simulink library "NexteerUtilities"  (R2013b)
settings: Solver=FixedStepDiscrete  StartTime=0.0  StopTime=10.0  FixedStep=.1  RelTol=1e-3
undefined symbols (not defined in the file or in its folder): CF_Uls_f32, LPF_Str
libraries: NexteerUtilities x5
settings Model: Creator=mmcbroom  LastModifiedBy=DZ1YRM

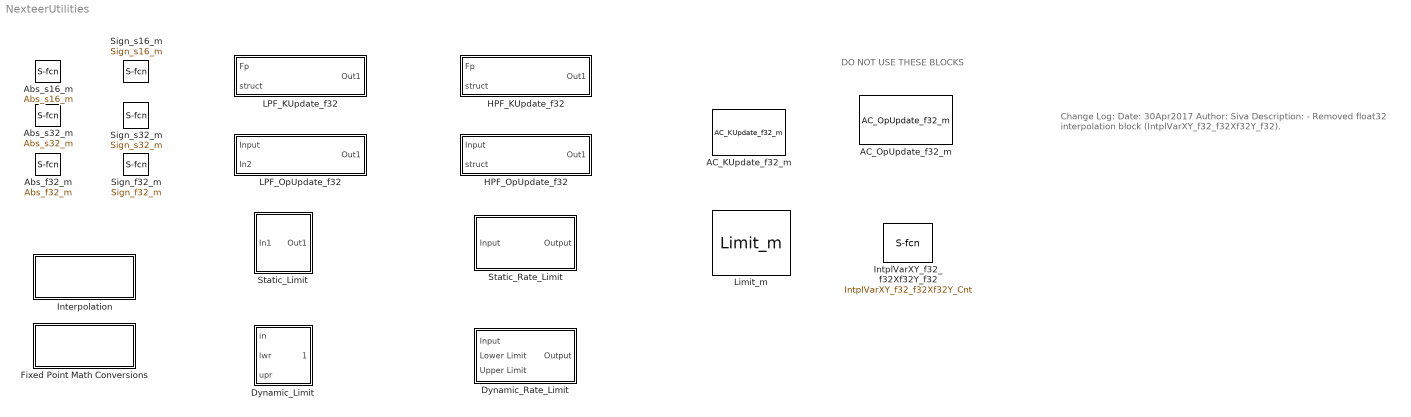
== system NexteerUtilities ==
  note: DO NOT USE THESE BLOCKS
  note: Change Log:
      |
      | Date: 30Apr2017
      | Author: Siva
      | Description:
      |      -  Removed float32 interpolation block (IntplVarXY_f32_f32Xf32Y_f32).
  AC_KUpdate_f32_m : S-Function  FunctionName=AC_KUpdate_f32_m  EnableBusSupport=off  mask(Legacy Function){}
      mask help:
      | This block allows you to call the legacy functions specified by the following Legacy Code Tool definition:
      | def.SFunctionName = 'util_LPF_KUpdate_f32';
      | def.OutputFcnSpec = 'single y1 = LPF_KUpdate_f32_m(single u1, single u2)';
      | def.HeaderFiles = {'utility.h'};
      | def.SourceFiles = {'utility.c'};
      settings: AttributesFormatString=Filt_KUpdate_f32
      mask Help: <p>This block was generated automatically by the Legacy Code Tool. For detailed help on this tool, call<a href="matlab:legacy_code('help')"> legacy_code('help')</a>.</p>
      mask Display:
      | port_label('input',1,'Fp');
      | port_label('input',2,'T');
      | port_label('output',1,'K');
      | 
      | text(0.3,0.5,'Do Not\n Use\nThis Block')
  AC_OpUpdate_f32_m : S-Function  FunctionName=AC_OpUpdate_f32_m  EnableBusSupport=off
      mask Display:
      | port_label('input',1,'in')
      | port_label('input',2,'PrevOut')
      | port_label('input',3,'K')
      | 
      | port_label('output',1,'out')
      | 
      | text(0.45,0.5,'Do Not\n Use\nThis Block')
  Abs_f32_m : S-Function  FunctionName=Abs_f32_m  EnableBusSupport=off  mask(Abs_f32){}
      mask help:
      | This block allows you to call the legacy functions specified by the following Legacy Code Tool definition:
      | def.SFunctionName = 'util_abs_f32';
      | def.OutputFcnSpec = 'single y1 = Abs_f32_m(single u1)';
      | def.HeaderFiles = {'utility.h'};
      settings: AttributesFormatString=Abs_f32
      mask Help: <p>This block was generated automatically by the Legacy Code Tool. For detailed help on this tool, call<a href="matlab:legacy_code('help')"> legacy_code('help')</a>.</p>
      mask Display:
      | fprintf('|u|');
      | %port_label('input',1,'U');
      | %port_label('output',1,'Y');
  Abs_s16_m : S-Function  FunctionName=Abs_s16_m  EnableBusSupport=off  mask(Abs_s16){}
      mask help:
      | This block allows you to call the legacy functions specified by the following Legacy Code Tool definition:
      | def.SFunctionName = 'util_abs_s16';
      | def.OutputFcnSpec = 'uint16 y1 = Abs_s16_m(int16 u1)';
      | def.HeaderFiles = {'utility.h'};
      settings: AttributesFormatString=Abs_s16
      mask Help: <p>This block was generated automatically by the Legacy Code Tool. For detailed help on this tool, call<a href="matlab:legacy_code('help')"> legacy_code('help')</a>.</p>
      mask Display:
      | fprintf('|u|');
      | %port_label('input',1,'s16');
      | %port_label('output',1,'Y');
  Abs_s32_m : S-Function  FunctionName=Abs_s32_m  EnableBusSupport=off  mask(Abs_s32){}
      mask help:
      | This block allows you to call the legacy functions specified by the following Legacy Code Tool definition:
      | def.SFunctionName = 'util_abs_s32';
      | def.OutputFcnSpec = 'uint32 y1 = Abs_s32_m(int32 u1)';
      | def.HeaderFiles = {'utility.h'};
      settings: AttributesFormatString=Abs_s32
      mask Help: <p>This block was generated automatically by the Legacy Code Tool. For detailed help on this tool, call<a href="matlab:legacy_code('help')"> legacy_code('help')</a>.</p>
      mask Display:
      | fprintf('|u|');
      | %port_label('input',1,'U');
      | %port_label('output',1,'Y');
  Dynamic_Limit : Subsystem  mask(Dynamic_Limit){}
      mask help: Simulink implementation of the Limit_m macro. This implementation allows the user to dynamically change the limit values.
      mask Display:
      | horizX = [0.2 0.9];
      | horizY = [0.55 0.55];
      | 
      | vertX = [0.55 0.55];
      | vertY = [0.2 0.8];
      | 
      | x = [.25, .35, .75, .85];
      | y = [.2, .2, .8, .8];
      | 
      | plot(horizX,horizY, vertX,vertY, x,y);
      | 
      | text(0.5,0.9,'f32', 'horizontalAlignment', 'center')
  Dynamic_Rate_Limit : Subsystem  mask(Dynamic_Rate_Limit){Ts=0}
      mask prompts: Ts "Time Step"
      mask help: Dynamic_Rate_Limit is a rate limiter with dynamic bounds.
      settings: AttributesFormatString=Time Step: %<Ts>
  Fixed Point Math Conversions : Subsystem
  HPF_KUpdate_f32 : Subsystem  mask(HPF_KUpdate_f32){Ts=0}
      mask prompts: Ts "Time Step"
      mask help: Simulink implementation of the HPF_KUpdate_f32_m macro.
      settings: AttributesFormatString=Time Step: %<Ts>
      mask Display:
      | port_label('input',1,'Hz');
      | port_label('input',2,'HPF_Str In');
      | port_label('output',1,'HPF_Str Out');
  HPF_OpUpdate_f32 : Subsystem  mask(HPF_OpUpdate_f32){}
      mask help: Simulink implementation of the HPF_OpUpdate_f32_m macro.
      mask Display:
      | port_label('input',1,'Input')
      | port_label('input',2,'HPF_Str In')
      | port_label('output',1,'HPF_Str Out')
  Interpolation : Subsystem
  IntplVarXY_f32_f32Xf32Y_f32 : S-Function  FunctionName=IntplVarXY_f32_f32Xf32Y_Cnt  Parameters=SParameter1, SParameter2  EnableBusSupport=off  mask(IntplVarXY_f32_f32Xf32Y_f32){SParameter1=ones([1 1 ]), SParameter2=ones([1 1 ])}
      mask prompts: SParameter1 "XTable:"; SParameter2 "YTable:"
      mask help:
      | This block allows you to call the legacy functions specified by the following Legacy Code Tool definition:
      | def.SFunctionName = 'IntplVarXY_f32_f32Xf32Y_Cnt';
      | def.OutputFcnSpec = 'single y1 = IntplVarXY_f32_f32Xf32Y_Cnt(single p1[], single p2[], uint16 size(p1,1), single u1)';
      | def.HeaderFiles = {'GlobalMacro.h'};
      | def.SourceFiles = {'utility.c'};
      settings: AttributesFormatString=IntplVarXY (float32)
      mask Help: <p>This block was generated automatically by the Legacy Code Tool. For detailed help on this tool, call<a href="matlab:legacy_code('help')"> legacy_code('help')</a>.</p>
      mask Display:
      | fprintf('float32\n\nInterpolate')
      | 
      | Xx = [0.1, .9];
      | Xy = [0.5, 0.5];
      | Yx = [0.5, 0.5];
      | Yy = [0.1, .8];
      | 
      | px = [.1, .3, .6, .7, .8, .9];
      | py = [.34,  .35, .39, .4, .5, .8];
      | plot(Xx,Xy, Yx,Yy, px,py)
  LPF_KUpdate_f32 : Subsystem  mask(LPF_KUpdate_f32){Ts=0}
      mask prompts: Ts "Time Step:"
      mask help: Simulink implementation of the LPF_KUpdate_f32_m macro.
      settings: AttributesFormatString=Time Step: %<Ts>
      mask Display:
      | port_label('input',1,'Hz');
      | port_label('input',2,'LPF_Str In');
      | port_label('output',1,'LPF_Str Out');
  LPF_OpUpdate_f32 : Subsystem  mask(LPF_OpUpdate_f32){}
      mask help: Simulink implementation of the LPF_OpUpdate_f32_m macro.
      mask Display:
      | port_label('input',1,'Input')
      | port_label('input',2,'LPF_Str In')
      | port_label('output',1,'LPF_Str Out')
  Limit_m : S-Function  FunctionName=Limit_m  EnableBusSupport=off
      mask help:
      | This block is being deprecated.
      | Use the Static_Limit or Dynamic_Limit blocks instead.
      settings: AttributesFormatString=%<Description>
      mask Display:
      | port_label('input',1,'U');
      | port_label('input',2,'Lower Limit');
      | port_label('input',3,'Upper Limit');
      | port_label('output',1,'Y');
      | text(0.3,0.76,'Do Not Use\nThis Block')
  Sign_f32_m : S-Function  FunctionName=Sign_f32_m  EnableBusSupport=off  mask(Sign_f32){}
      mask help:
      | This block allows you to call the legacy functions specified by the following Legacy Code Tool definition:
      | def.SFunctionName = 'util_sign_f32';
      | def.OutputFcnSpec = 'single y1 = Sign_f32_m(single u1)';
      | def.HeaderFiles = {'utility.h'};
      settings: AttributesFormatString=Sign_f32
      mask Help: <p>This block was generated automatically by the Legacy Code Tool. For detailed help on this tool, call<a href="matlab:legacy_code('help')"> legacy_code('help')</a>.</p>
      mask Display:
      | %port_label('input',1,'U');
      | %port_label('output',1,'Y');
      | 
      | Xx = [-1, 1];
      | Xy = [ 0, 0];
      | Yx = [ 0, 0];
      | Yy = [-1, 1];
      | 
      | px = [-.8, 0, 0, 0.8];
      | py = [-.4, -.4, .4, .4];
      | plot(Xx,Xy, Yx,Yy, px,py)
  Sign_s16_m : S-Function  FunctionName=Sign_s16_m  EnableBusSupport=off  mask(Sign_s16){}
      mask help:
      | This block allows you to call the legacy functions specified by the following Legacy Code Tool definition:
      | def.SFunctionName = 'util_sign_s16';
      | def.OutputFcnSpec = 'int16 y1 = Sign_s16_m(int16 u1)';
      | def.HeaderFiles = {'utility.h'};
      settings: AttributesFormatString=Sign_s16
      mask Help: <p>This block was generated automatically by the Legacy Code Tool. For detailed help on this tool, call<a href="matlab:legacy_code('help')"> legacy_code('help')</a>.</p>
      mask Display:
      | %port_label('input',1,'U');
      | %port_label('output',1,'Out');
      | 
      | Xx = [-1, 1];
      | Xy = [ 0, 0];
      | Yx = [ 0, 0];
      | Yy = [-1, 1];
      | 
      | px = [-.8, 0, 0, 0.8];
      | py = [-.4, -.4, .4, .4];
      | plot(Xx,Xy, Yx,Yy, px,py)
  Sign_s32_m : S-Function  FunctionName=Sign_s32_m  EnableBusSupport=off  mask(Sign_s32){}
      mask help:
      | This block allows you to call the legacy functions specified by the following Legacy Code Tool definition:
      | def.SFunctionName = 'util_sign_s32';
      | def.OutputFcnSpec = 'int32 y1 = Sign_s32_m(int32 u1)';
      | def.HeaderFiles = {'utility.h'};
      settings: AttributesFormatString=Sign_s32
      mask Help: <p>This block was generated automatically by the Legacy Code Tool. For detailed help on this tool, call<a href="matlab:legacy_code('help')"> legacy_code('help')</a>.</p>
      mask Display:
      | %port_label('input',1,'U');
      | %port_label('output',1,'Y');
      | 
      | Xx = [-1, 1];
      | Xy = [ 0, 0];
      | Yx = [ 0, 0];
      | Yy = [-1, 1];
      | 
      | px = [-.8, 0, 0, 0.8];
      | py = [-.4, -.4, .4, .4];
      | plot(Xx,Xy, Yx,Yy, px,py)
  Static_Limit : Subsystem  mask(Static_Limit){uprlim=0, lwrlim=0}
      mask prompts: uprlim "Upper Limit"; lwrlim "Lower Limit"
      mask help: Simulink implementation of the Limit_m macro. This implementation fixes limit values.
      settings: AttributesFormatString=|
      | Upper Limit:%<uprlim>
      | Lower Limit:%<lwrlim>
      mask Display:
      | horizX = [0.2 0.9];
      | horizY = [0.55 0.55];
      | 
      | vertX = [0.55 0.55];
      | vertY = [0.2 0.8];
      | 
      | x = [.25, .35, .75, .85];
      | y = [.2, .2, .8, .8];
      | 
      | plot(horizX,horizY, vertX,vertY, x,y);
      | 
      | text(0.5,0.9,'f32', 'horizontalAlignment', 'center')
  Static_Rate_Limit : Subsystem  mask(Static_Rate_Limit){Ts=0, LowerLimit=0, UpperLimit=0}
      mask prompts: Ts "Time Step"; LowerLimit "Lower Limit"; UpperLimit "Upper Limit"
      mask help: Static_Rate_Limit provides a rate limiter with static limit bounds.
      settings: AttributesFormatString=|
      | Time Step: %<Ts>
      | Lower Limit: %<LowerLimit>
      | Upper Limit: %<UpperLimit>

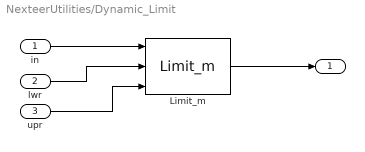
== system NexteerUtilities/Dynamic_Limit ==
  in : Inport
  lwr : Inport  Port=2
  upr : Inport  Port=3
  Limit_m : NexteerUtilities/Static_Limit/Limit_m
  " " : Outport
  wires:
  Limit_m/1 -> " "/1
  in/1 -> Limit_m/1
  lwr/1 -> Limit_m/2
  upr/1 -> Limit_m/3

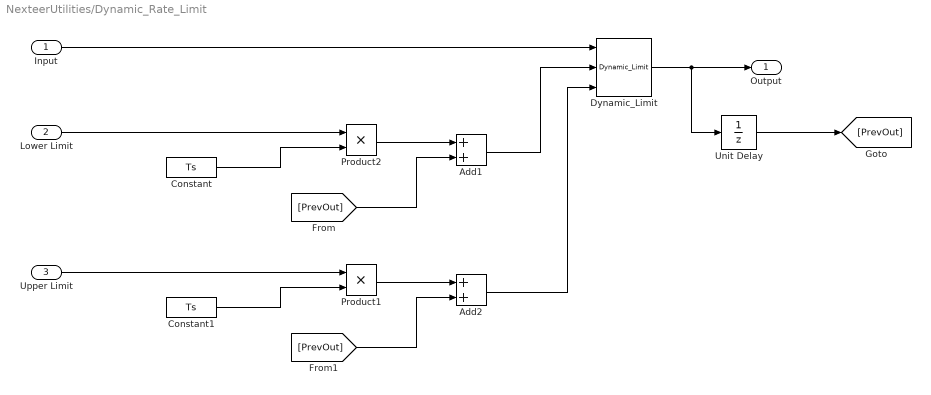
== system NexteerUtilities/Dynamic_Rate_Limit ==
  Input : Inport
  Lower Limit : Inport  Port=2
  Upper Limit : Inport  Port=3
  Add1 : Sum
  Add2 : Sum
  Constant : Constant  Value=Ts
  Constant1 : Constant  Value=Ts
  Dynamic_Limit : NexteerUtilities/Dynamic_Limit
  Product1 : Product
  Product2 : Product
  Unit Delay : UnitDelay  SampleTime=-1
  Output : Outport
  wires:
  Dynamic_Limit/1 -> Unit Delay/1, Output/1
  Input/1 -> Dynamic_Limit/1
  Constant/1 -> Product2/2
  Lower Limit/1 -> Product2/1
  Product2/1 -> Add1/1
  Unit Delay/1 -> [PrevOut]
  [PrevOut] -> Add1/2
  Constant1/1 -> Product1/2
  Upper Limit/1 -> Product1/1
  Product1/1 -> Add2/1
  [PrevOut] -> Add2/2
  Add1/1 -> Dynamic_Limit/2
  Add2/1 -> Dynamic_Limit/3

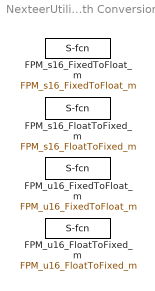
== system NexteerUtilities/Fixed Point Math Conversions ==
  FPM_s16_FixedToFloat_m : S-Function  FunctionName=FPM_s16_FixedToFloat_m  Parameters=SParameter1  EnableBusSupport=off  mask(s16_FixedToFloat){SFunctionSpec=single y1 = FPM_s16_FixedToFloat_m(int16 u1,  single p1), Param1=1}
      mask prompts: Param1 "P1:"
      mask help:
      | This block allows you to call the legacy functions specified by the following Legacy Code Tool definition:
      | def.SFunctionName = 'FPM_s16_FixedToFloat_m';
      | def.OutputFcnSpec = 'single y1 = FPM_s16_FixedToFloat_m(int16 u1,  single p1)';
      | def.HeaderFiles = {'GlobalMacro.h', 'fixmath.h'};
      | def.SourceFiles = {'utility.c'};
      | def.IncPaths = {'..'};
      | def.SrcPaths = {'..'};
      mask init:
      | SParameter1 = 2^-Param1;
      settings: AttributesFormatString=s16_FixedToFloat
      mask Help: <p>This block was generated automatically by the Legacy Code Tool. For detailed help on this tool, call<a href="matlab:legacy_code('help')"> legacy_code('help')</a>.</p>
      mask Display:
      | pnum = Param1;
      | unum = 15-Param1;
      | 
      | port_label('output',1,'f32')
      | 
      | if pnum<0
      |    fptxt = ['s' num2str(unum) 'pm' num2str(abs(pnum))];
      |    %fprintf(['s' num2str(unum) 'pm' num2str(abs(pnum))]);
      | elseif pnum>15
      |    fptxt = ['sm' num2str(abs(unum)) 'p' num2str(pnum)];
      |    %fprintf(['sm' num2str(abs(unum)) 'p' num2str(pnum)]);
      | else
      |    fptxt = ['s' num2str(unum) 'p' num2str(pnum)];
      |    %fprintf(['s' num2str(unum) 'p' num2str(pnum)]);
      | end
      | 
      | port_label('input',1,fptxt)
  FPM_s16_FloatToFixed_m : S-Function  FunctionName=FPM_s16_FloatToFixed_m  Parameters=SParameter1  EnableBusSupport=off  mask(s16_FloatToFixed){SFunctionSpec=int16  y1 = FPM_s16_FloatToFixed_m(single u1, single p1), Param1=1}
      mask prompts: Param1 "P1:"
      mask help:
      | This block allows you to call the legacy functions specified by the following Legacy Code Tool definition:
      | def.SFunctionName = 'FPM_s16_FloatToFixed_m';
      | def.OutputFcnSpec = 'int16  y1 = FPM_s16_FloatToFixed_m(single u1, single p1)';
      | def.HeaderFiles = {'GlobalMacro.h', 'fixmath.h'};
      | def.SourceFiles = {'utility.c'};
      | def.IncPaths = {'..'};
      | def.SrcPaths = {'..'};
      mask init:
      | SParameter1 = 2^Param1;
      settings: AttributesFormatString=s16_FloatToFixed
      mask Help: <p>This block was generated automatically by the Legacy Code Tool. For detailed help on this tool, call<a href="matlab:legacy_code('help')"> legacy_code('help')</a>.</p>
      mask Display:
      | pnum = Param1;
      | unum = 15-Param1;
      | 
      | port_label('input',1,'f32')
      | 
      | if pnum<0
      |     fptxt = ['s' num2str(unum) 'pm' num2str(abs(pnum))];
      |     %fprintf(['s' num2str(unum) 'pm' num2str(abs(pnum))]);
      | elseif pnum>15
      |     fptxt = ['sm' num2str(abs(unum)) 'p' num2str(pnum)];
      |     %fprintf(['sm' num2str(abs(unum)) 'p' num2str(pnum)]);
      | else
      |     fptxt = ['s' num2str(unum) 'p' num2str(pnum)];
      |     %fprintf(['s' num2str(unum) 'p' num2str(pnum)]);
      | end
      | 
      | port_label('output',1,fptxt)
  FPM_u16_FixedToFloat_m : S-Function  FunctionName=FPM_u16_FixedToFloat_m  Parameters=SParameter1  EnableBusSupport=off  mask(u16_FixedToFloat){SFunctionSpec=single y1 = FPM_u16_FixedToFloat_m(uint16 u1, single p1), Param1=1}
      mask prompts: Param1 "P1:"
      mask help:
      | This block allows you to call the legacy functions specified by the following Legacy Code Tool definition:
      | def.SFunctionName = 'FPM_u16_FixedToFloat_m';
      | def.OutputFcnSpec = 'single y1 = FPM_u16_FixedToFloat_m(uint16 u1, single p1)';
      | def.HeaderFiles = {'GlobalMacro.h', 'fixmath.h'};
      | def.SourceFiles = {'utility.c'};
      | def.IncPaths = {'..'};
      | def.SrcPaths = {'..'};
      mask init:
      | SParameter1 = 2^-Param1;
      settings: AttributesFormatString=u16_FixedToFloat
      mask Help: <p>This block was generated automatically by the Legacy Code Tool. For detailed help on this tool, call<a href="matlab:legacy_code('help')"> legacy_code('help')</a>.</p>
      mask Display:
      | pnum = Param1;
      | unum = 16-Param1;
      | 
      | port_label('output',1,'f32')
      | 
      | if pnum<0
      |    fptxt =  ['u' num2str(unum) 'pm' num2str(abs(pnum))];
      |    %fprintf(['u' num2str(unum) 'pm' num2str(abs(pnum))]);
      | elseif pnum>16
      |    fptxt = ['um' num2str(abs(unum)) 'p' num2str(pnum)];
      |    %fprintf(['um' num2str(abs(unum)) 'p' num2str(pnum)]);
      | else
      |    fptxt = ['u' num2str(unum) 'p' num2str(pnum)];
      |    %fprintf(['u' num2str(unum) 'p' num2str(pnum)]);
      | end
      | 
      | port_label('input',1,fptxt)
  FPM_u16_FloatToFixed_m : S-Function  FunctionName=FPM_u16_FloatToFixed_m  Parameters=SParameter1  EnableBusSupport=off  mask(u16_FloatToFixed){SFunctionSpec=uint16 y1 = FPM_u16_FloatToFixed_m(single u1, single p1), Param1=1}
      mask prompts: Param1 "P1:"
      mask help:
      | This block allows you to call the legacy functions specified by the following Legacy Code Tool definition:
      | def.SFunctionName = 'FPM_u16_FloatToFixed_m';
      | def.OutputFcnSpec = 'uint16 y1 = FPM_u16_FloatToFixed_m(single u1, single p1)';
      | def.HeaderFiles = {'GlobalMacro.h', 'fixmath.h'};
      | def.SourceFiles = {'utility.c'};
      | def.IncPaths = {'..'};
      | def.SrcPaths = {'..'};
      mask init:
      | SParameter1 = 2^Param1;
      settings: AttributesFormatString=u16_FloatToFixed
      mask Help: <p>This block was generated automatically by the Legacy Code Tool. For detailed help on this tool, call<a href="matlab:legacy_code('help')"> legacy_code('help')</a>.</p>
      mask Display:
      | pnum = Param1;
      | 
      | unum = 16-Param1;
      | 
      | port_label('input',1,'f32')
      | 
      | if pnum<0
      |     fptxt = ['u' num2str(unum) 'pm' num2str(abs(pnum))];
      |     %fprintf(['f32 ---> ' 'u' num2str(unum) 'pm' num2str(abs(pnum))]);
      | elseif pnum>16
      |     fptxt = ['um' num2str(abs(unum)) 'p' num2str(pnum)];
      |     %fprintf(['f32 ---> ' 'um' num2str(abs(unum)) 'p' num2str(pnum)]);
      | else
      |     fptxt = ['u' num2str(unum) 'p' num2str(pnum)];
      |     %fprintf(['f32 ---> ' 'u' num2str(unum) 'p' num2str(pnum)]);
      | end
      | 
      | port_label('output',1,fptxt)

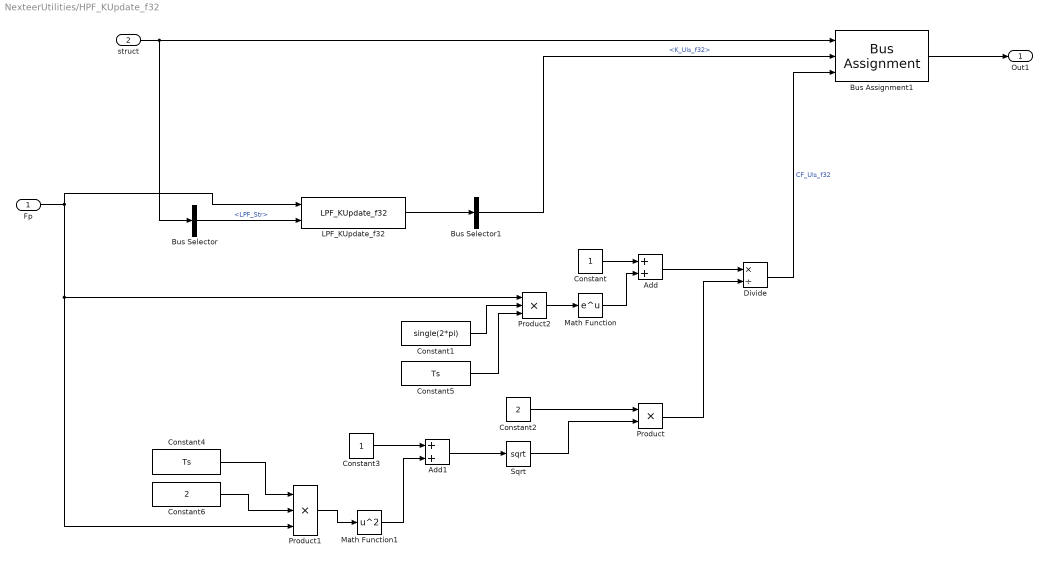
== system NexteerUtilities/HPF_KUpdate_f32 ==
  Fp : Inport
  struct : Inport  Port=2  OutDataTypeStr=Bus: HPF32KSV_Str
  Add : Sum
  Add1 : Sum
  Bus Assignment1 : BusAssignment  AssignedSignals=LPF_Str.K_Uls_f32,CF_Uls_f32
  Bus Selector : BusSelector  OutputSignals=LPF_Str
  Bus Selector1 : BusSelector  OutputSignals=K_Uls_f32
  Constant : Constant  OutDataTypeStr=single
  Constant1 : Constant  Value=single(2*pi)  OutDataTypeStr=single
  Constant2 : Constant  Value=2  OutDataTypeStr=single
  Constant3 : Constant  OutDataTypeStr=single
  Constant4 : Constant  Value=Ts  OutDataTypeStr=single
  Constant5 : Constant  Value=Ts  OutDataTypeStr=single
  Constant6 : Constant  Value=2  OutDataTypeStr=single
  Divide : Product  Inputs=*/
  LPF_KUpdate_f32 : NexteerUtilities/LPF_KUpdate_f32  Ts=Ts
  Math Function : Math  SaturateOnIntegerOverflow=on
  Math Function1 : Math  Operator=square  SaturateOnIntegerOverflow=on
  Product : Product
  Product1 : Product  Inputs=3
  Product2 : Product  Inputs=3
  Sqrt : Sqrt  SaturateOnIntegerOverflow=on
  Out1 : Outport  OutDataTypeStr=Bus: HPF32KSV_Str
  wires:
  Fp/1 -> LPF_KUpdate_f32/1, Product1/3, Product2/1
  struct/1 -> Bus Selector/1, Bus Assignment1/1
  Constant/1 -> Add/1
  Constant1/1 -> Product2/2
  Math Function/1 -> Add/2
  Add/1 -> Divide/1
  Sqrt/1 -> Product/2
  Constant2/1 -> Product/1
  Constant3/1 -> Add1/1
  Add1/1 -> Sqrt/1
  Constant4/1 -> Product1/1
  Product/1 -> Divide/2
  Product2/1 -> Math Function/1
  Math Function1/1 -> Add1/2
  Product1/1 -> Math Function1/1
  Bus Assignment1/1 -> Out1/1
  LPF_KUpdate_f32/1 -> Bus Selector1/1
  Divide/1 -> Bus Assignment1/3  "CF_Uls_f32"
  Bus Selector/1 -> LPF_KUpdate_f32/2  "<LPF_Str>"
  Bus Selector1/1 -> Bus Assignment1/2  "<K_Uls_f32>"
  Constant5/1 -> Product2/3
  Constant6/1 -> Product1/2

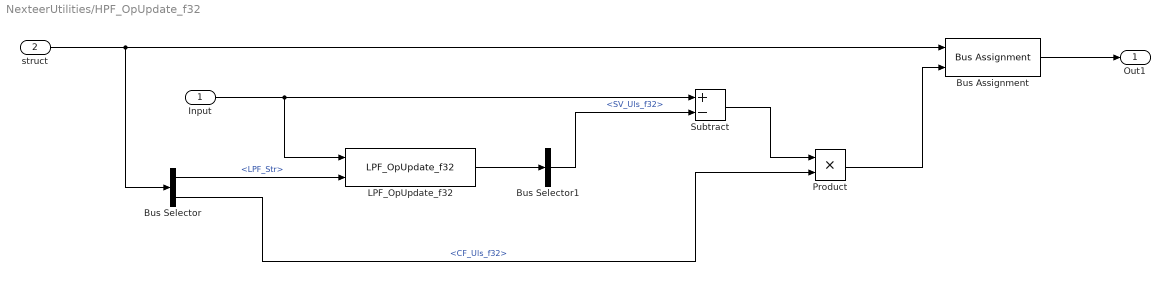
== system NexteerUtilities/HPF_OpUpdate_f32 ==
  Input : Inport
  struct : Inport  Port=2  OutDataTypeStr=Bus: HPF32KSV_Str
  Bus Assignment : BusAssignment  AssignedSignals=LPF_Str.SV_Uls_f32
  Bus Selector : BusSelector  OutputSignals=LPF_Str,CF_Uls_f32
  Bus Selector1 : BusSelector  OutputSignals=SV_Uls_f32
  LPF_OpUpdate_f32 : NexteerUtilities/LPF_OpUpdate_f32
  Product : Product
  Subtract : Sum  Inputs=+-
  Out1 : Outport  OutDataTypeStr=Bus: HPF32KSV_Str
  wires:
  struct/1 -> Bus Selector/1, Bus Assignment/1
  Bus Selector/1 -> LPF_OpUpdate_f32/2  "<LPF_Str>"
  LPF_OpUpdate_f32/1 -> Bus Selector1/1
  Input/1 -> LPF_OpUpdate_f32/1, Subtract/1
  Bus Selector1/1 -> Subtract/2  "<SV_Uls_f32>"
  Bus Selector/2 -> Product/2  "<CF_Uls_f32>"
  Subtract/1 -> Product/1
  Product/1 -> Bus Assignment/2
  Bus Assignment/1 -> Out1/1

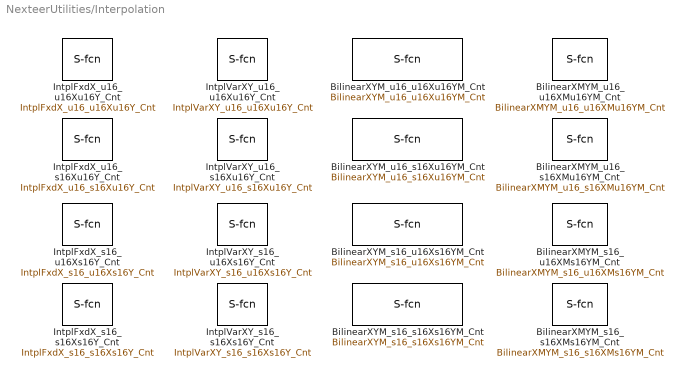
== system NexteerUtilities/Interpolation ==
  BilinearXMYM_s16_s16XMs16YM_Cnt : S-Function  FunctionName=BilinearXMYM_s16_s16XMs16YM_Cnt  Parameters=Param1,Param2,Param3  EnableBusSupport=off  mask(BilinearXMYM_s16_s16XMs16YM_Cnt){Param1=0, Param2=0, Param3=0}
      mask prompts: Param1 "BSTable:"; Param2 "XMTable:"; Param3 "YMTable:"
      settings: AttributesFormatString=Bilinear (sXM, sYM)
      mask Help: <p>This block was generated automatically by the Legacy Code Tool. For detailed help on this tool, call<a href="matlab:legacy_code('help')"> legacy_code('help')</a>.</p>
      mask Display:
      | port_label('input',1,'BS');
      | port_label('input',2,'u');
      | %port_label('output',1,'y');
      | 
      | Xx = [0.1, .9];
      | Xy = [0.5, 0.5];
      | Yx = [0.5, 0.5];
      | Yy = [0.1, .9];
      | 
      | px = [.15, .3, .6, .7, .8, .9];
      | py1 = [.1,  .1, .3, .4, .5, .9];
      | py2 = py1+0.15;
      | py3 = py2+0.15;
      | plot(Xx,Xy, Yx,Yy, px,py1, px,py2, px,py3)
  BilinearXMYM_s16_u16XMs16YM_Cnt : S-Function  FunctionName=BilinearXMYM_s16_u16XMs16YM_Cnt  Parameters=Param1,Param2,Param3  EnableBusSupport=off  mask(BilinearXMYM_s16_u16XMs16YM_Cnt){Param1=0, Param2=0, Param3=0}
      mask prompts: Param1 "BSTable:"; Param2 "XMTable:"; Param3 "YMTable:"
      settings: AttributesFormatString=Bilinear (uXM, sXM)
      mask Help: <p>This block was generated automatically by the Legacy Code Tool. For detailed help on this tool, call<a href="matlab:legacy_code('help')"> legacy_code('help')</a>.</p>
      mask Display:
      | port_label('input',1,'BS');
      | port_label('input',2,'u');
      | %port_label('output',1,'y');
      | 
      | Xx = [0.2, .9];
      | Xy = [0.4, 0.4];
      | Yx = [0.2, 0.2];
      | Yy = [0, .7];
      | 
      | px = [0.2, .3, .4, .6, .8, .9];
      | py1 = [.72, .7, .6, .3, .25, .25];
      | py2 = py1-0.1;
      | py3 = py2-0.1;
      | 
      | plot(Xx,Xy, Yx,Yy, px,py1, px,py2, px,py3)
  BilinearXMYM_u16_s16XMu16YM_Cnt : S-Function  FunctionName=BilinearXMYM_u16_s16XMu16YM_Cnt  Parameters=Param1,Param2,Param3  EnableBusSupport=off  mask(BilinearXMYM_u16_s16XMu16YM_Cnt){Param1=0, Param2=0, Param3=0}
      mask prompts: Param1 "BSTable:"; Param2 "XMTable:"; Param3 "YMTable:"
      settings: AttributesFormatString=Bilinear (sXM, uYM)
      mask Help: <p>This block was generated automatically by the Legacy Code Tool. For detailed help on this tool, call<a href="matlab:legacy_code('help')"> legacy_code('help')</a>.</p>
      mask Display:
      | port_label('input',1,'BS');
      | port_label('input',2,'u');
      | %port_label('output',1,'y');
      | 
      | Xx = [0, .9];
      | Xy = [.05, .05];
      | Yx = [.45, .45];
      | Yy = [.05, .9];
      | 
      | px = [0.15, .3, .4, .6, .7, .9];
      | py1 = [.1, .1, .2, .5, .6, .65];
      | py2 = py1+.15;
      | py3 = py2+.15;
      | 
      | plot(Xx,Xy, Yx,Yy, px,py1, px,py2, px,py3)
  BilinearXMYM_u16_u16XMu16YM_Cnt : S-Function  FunctionName=BilinearXMYM_u16_u16XMu16YM_Cnt  Parameters=Param1,Param2,Param3  EnableBusSupport=off  mask(BilinearXMYM_u16_u16XMu16YM_Cnt){Param1=0, Param2=0, Param3=0}
      mask prompts: Param1 "BSTable:"; Param2 "XMTable:"; Param3 "YMTable:"
      settings: AttributesFormatString=Bilinear (uXM, uYM)
      mask Help: <p>This block was generated automatically by the Legacy Code Tool. For detailed help on this tool, call<a href="matlab:legacy_code('help')"> legacy_code('help')</a>.</p>
      mask Display:
      | port_label('input',1,'BS');
      | port_label('input',2,'u');
      | %port_label('output',1,'y');
      | 
      | Xx = [0.2, .9];
      | Xy = [0.1, 0.1];
      | Yx = [0.2, 0.2];
      | Yy = [0.1, .7];
      | 
      | px = [0.2, .3, .4, .5, .6, .7, .9];
      | 
      | py1 = [0.1,  0.4, .6, .7, .75, .8, .8];
      | py2 = [0.1,  0.4, .5, .6, .65, .7, .7];
      | py3 = [0.1,  0.3, .4, .5, .55, .6, .6];
      | 
      | plot(Xx,Xy, Yx,Yy, px,py1, px,py2, px,py3)
  BilinearXYM_s16_s16Xs16YM_Cnt : S-Function  FunctionName=BilinearXYM_s16_s16Xs16YM_Cnt  Parameters=Param1,Param2,Param3  EnableBusSupport=off  mask(BilinearXYM_s16_s16Xs16YM_Cnt){Param1=0, Param2=0, Param3=0}
      mask prompts: Param1 "BSTable:"; Param2 "XTable:"; Param3 "YMTable:"
      settings: AttributesFormatString=Bilinear (sX, xYM)
      mask Help: <p>This block was generated automatically by the Legacy Code Tool. For detailed help on this tool, call<a href="matlab:legacy_code('help')"> legacy_code('help')</a>.</p>
      mask Display:
      | port_label('input',1,'BS');
      | port_label('input',2,'u');
      | %port_label('output',1,'y');
      | 
      | fprintf('   Bilinear Interp\n   X-tbl: s16 vector\n   Y-tbl: s16 matrix')
  BilinearXYM_s16_u16Xs16YM_Cnt : S-Function  FunctionName=BilinearXYM_s16_u16Xs16YM_Cnt  Parameters=Param1,Param2,Param3  EnableBusSupport=off  mask(BilinearXYM_s16_u16Xs16YM_Cnt){Param1=0, Param2=0, Param3=0}
      mask prompts: Param1 "BSTable:"; Param2 "XTable:"; Param3 "YMTable:"
      settings: AttributesFormatString=Bilinear (uX, sYM)
      mask Help: <p>This block was generated automatically by the Legacy Code Tool. For detailed help on this tool, call<a href="matlab:legacy_code('help')"> legacy_code('help')</a>.</p>
      mask Display:
      | port_label('input',1,'BS');
      | port_label('input',2,'u');
      | %port_label('output',1,'y');
      | 
      | fprintf('   Bilinear Interp\n   X-tbl: u16 vector\n   Y-tbl: s16 matrix')
  BilinearXYM_u16_s16Xu16YM_Cnt : S-Function  FunctionName=BilinearXYM_u16_s16Xu16YM_Cnt  Parameters=Param1,Param2,Param3  EnableBusSupport=off  mask(BilinearXYM_u16_s16Xu16YM_Cnt){Param1=0, Param2=0, Param3=0}
      mask prompts: Param1 "BSTable:"; Param2 "XTable:"; Param3 "YMTable:"
      settings: AttributesFormatString=Bilinear (sX, uYM)
      mask Help: <p>This block was generated automatically by the Legacy Code Tool. For detailed help on this tool, call<a href="matlab:legacy_code('help')"> legacy_code('help')</a>.</p>
      mask Display:
      | port_label('input',1,'BS');
      | port_label('input',2,'u');
      | %port_label('output',1,'y');
      | 
      | fprintf('   Bilinear Interp\n   X-tbl: s16 vector\n   Y-tbl: u16 matrix')
  BilinearXYM_u16_u16Xu16YM_Cnt : S-Function  FunctionName=BilinearXYM_u16_u16Xu16YM_Cnt  Parameters=Param1,Param2,Param3  EnableBusSupport=off  mask(BilinearXYM_u16_u16Xu16YM_Cnt){Param1=0, Param2=0, Param3=0}
      mask prompts: Param1 "BSTable:"; Param2 "XTable:"; Param3 "YMTable:"
      settings: AttributesFormatString=Bilinear (uX, uYM)
      mask Help: <p>This block was generated automatically by the Legacy Code Tool. For detailed help on this tool, call<a href="matlab:legacy_code('help')"> legacy_code('help')</a>.</p>
      mask Display:
      | port_label('input',1,'BS');
      | port_label('input',2,'u');
      | %port_label('output',1,'y');
      | 
      | fprintf('   Bilinear Interp\n   X-tbl: u16 vector\n   Y-tbl: u16 matrix')
  IntplFxdX_s16_s16Xs16Y_Cnt : S-Function  FunctionName=IntplFxdX_s16_s16Xs16Y_Cnt  Parameters=Param1,Param2  EnableBusSupport=off  mask(IntplFxdX_s16_s16Xs16Y_Cnt){Param1=0, Param2=0}
      mask prompts: Param1 "DelatX:"; Param2 "YTable:"
      settings: AttributesFormatString=IntplFxd (sX, sY)
      mask Help: <p>This block was generated automatically by the Legacy Code Tool. For detailed help on this tool, call<a href="matlab:legacy_code('help')"> legacy_code('help')</a>.</p>
      mask Display:
      | Xx = [0.1, .9];
      | Xy = [0.5, 0.5];
      | Yx = [0.5, 0.5];
      | Yy = [0.1, .9];
      | 
      | px = [.1, .3, .6, .7, .8, .9];
      | py = [.1,  .1, .3, .4, .5, .9];
      | 
      | %tic marks
      | tx1 = [0.2, 0.2];
      | tx2 = tx1 + 0.15;
      | tx3 = tx2 + 0.15;
      | tx4 = tx3 + 0.15;
      | tx5 = tx4 + 0.15;
      | ty = [.4, .6];
      | 
      | plot(Xx,Xy, Yx,Yy, px,py, tx1,ty, tx2,ty, tx3,ty, tx4,ty, tx5,ty)
  IntplFxdX_s16_u16Xs16Y_Cnt : S-Function  FunctionName=IntplFxdX_s16_u16Xs16Y_Cnt  Parameters=Param1,Param2  EnableBusSupport=off  mask(IntplFxdX_s16_u16Xs16Y_Cnt){Param1=0, Param2=0}
      mask prompts: Param1 "DelatX:"; Param2 "YTable:"
      settings: AttributesFormatString=IntplFxd (uX, sY)
      mask Help: <p>This block was generated automatically by the Legacy Code Tool. For detailed help on this tool, call<a href="matlab:legacy_code('help')"> legacy_code('help')</a>.</p>
      mask Display:
      | Xx = [0.1, .9];
      | Xy = [0.4, 0.4];
      | Yx = [0.1, 0.1];
      | Yy = [0, .9];
      | 
      | px = [0.1, .2, .3, .5, .7, .9];
      | py = [.75, .75, .6, .3, .1, .1];
      | 
      | %tic marks
      | tx1 = [0.2, 0.2];
      | tx2 = tx1 + 0.15;
      | tx3 = tx2 + 0.15;
      | tx4 = tx3 + 0.15;
      | tx5 = tx4 + 0.15;
      | ty = [.27, .53];
      | 
      | plot(Xx,Xy, Yx,Yy, px,py, tx1,ty, tx2,ty, tx3,ty, tx4,ty, tx5,ty)
  IntplFxdX_u16_s16Xu16Y_Cnt : S-Function  FunctionName=IntplFxdX_u16_s16Xu16Y_Cnt  Parameters=Param1,Param2  EnableBusSupport=off  mask(IntplFxdX_u16_s16Xu16Y_Cnt){Param1=0, Param2=0}
      mask prompts: Param1 "DelatX:"; Param2 "YTable:"
      settings: AttributesFormatString=IntplFxd (sX, uY)
      mask Help: <p>This block was generated automatically by the Legacy Code Tool. For detailed help on this tool, call<a href="matlab:legacy_code('help')"> legacy_code('help')</a>.</p>
      mask Display:
      | Xx = [0, .9];
      | Xy = [.05, .05];
      | Yx = [.45, .45];
      | Yy = [.05, .9];
      | 
      | px = [0, .3, .4, .6, .7, .9];
      | py = [.15, .15, .2, .5, .6, .65];
      | 
      | %tic marks
      | tx1 = [0.2, 0.2];
      | tx2 = tx1 + 0.15;
      | tx3 = tx2 + 0.15;
      | tx4 = tx3 + 0.15;
      | tx5 = tx4 + 0.15;
      | ty = [.1, .25];
      | 
      | plot(Xx,Xy, Yx,Yy, px,py, tx1,ty, tx2,ty, tx3,ty, tx4,ty, tx5,ty)
  IntplFxdX_u16_u16Xu16Y_Cnt : S-Function  FunctionName=IntplFxdX_u16_u16Xu16Y_Cnt  Parameters=Param1,Param2  EnableBusSupport=off  mask(IntplFxdX_u16_u16Xu16Y_Cnt){Param1=0, Param2=0}
      mask prompts: Param1 "DelatX:"; Param2 "YTable:"
      settings: AttributesFormatString=IntplFxd (uX, uY)
      mask Help: <p>This block was generated automatically by the Legacy Code Tool. For detailed help on this tool, call<a href="matlab:legacy_code('help')"> legacy_code('help')</a>.</p>
      mask Display:
      | %port_label('input',1,'u');
      | %port_label('output',1,'y');
      | 
      | Xx = [0.1, .9];
      | Xy = [0.1, 0.1];
      | Yx = [0.1, 0.1];
      | Yy = [0.1, .9];
      | 
      | px = [0.1, .2, .3, .4, .5, .6, .8];
      | py = [0.1,  0.4, .6, .7, .75, .78, .8];
      | 
      | %tic marks
      | tx1 = [0.2, 0.2];
      | tx2 = tx1 + 0.15;
      | tx3 = tx2 + 0.15;
      | tx4 = tx3 + 0.15;
      | tx5 = tx4 + 0.15;
      | ty = [.1, .25];
      | 
      | plot(Xx,Xy, Yx,Yy, px,py, tx1,ty, tx2,ty, tx3,ty, tx4,ty, tx5,ty)
  IntplVarXY_s16_s16Xs16Y_Cnt : S-Function  FunctionName=IntplVarXY_s16_s16Xs16Y_Cnt  Parameters=Param1,Param2  EnableBusSupport=off  mask(IntplVarXY_s16_s16Xs16Y_Cnt){Param1=0, Param2=0}
      mask prompts: Param1 "XTable:"; Param2 "YTable:"
      settings: AttributesFormatString=IntplVarXY (sX, sY)
      mask Help: <p>This block was generated automatically by the Legacy Code Tool. For detailed help on this tool, call<a href="matlab:legacy_code('help')"> legacy_code('help')</a>.</p>
      mask Display:
      | %port_label('input',1,'u');
      | %port_label('output',1,'(s16)');
      | 
      | Xx = [0.1, .9];
      | Xy = [0.5, 0.5];
      | Yx = [0.5, 0.5];
      | Yy = [0.1, .9];
      | 
      | px = [.1, .3, .6, .7, .8, .9];
      | py = [.1,  .1, .3, .4, .5, .9];
      | plot(Xx,Xy, Yx,Yy, px,py)
  IntplVarXY_s16_u16Xs16Y_Cnt : S-Function  FunctionName=IntplVarXY_s16_u16Xs16Y_Cnt  Parameters=Param1,Param2  EnableBusSupport=off  mask(IntplVarXY_s16_u16Xs16Y_Cnt){Param1=0, Param2=0}
      mask prompts: Param1 "XTable:"; Param2 "YTable:"
      settings: AttributesFormatString=IntplVarXY (uX, sY)
      mask Help: <p>This block was generated automatically by the Legacy Code Tool. For detailed help on this tool, call<a href="matlab:legacy_code('help')"> legacy_code('help')</a>.</p>
      mask Display:
      | %port_label('input',1,'u');
      | %port_label('output',1,'(s16)');
      | 
      | Xx = [0.1, .9];
      | Xy = [0.4, 0.4];
      | Yx = [0.1, 0.1];
      | Yy = [0, .9];
      | 
      | px = [0.1, .2, .3, .5, .7, .9];
      | py = [.75, .75, .6, .3, .1, .1];
      | plot(Xx,Xy, Yx,Yy, px,py)
  IntplVarXY_u16_s16Xu16Y_Cnt : S-Function  FunctionName=IntplVarXY_u16_s16Xu16Y_Cnt  Parameters=Param1,Param2  EnableBusSupport=off  mask(IntplVarXY_u16_s16Xu16Y_Cnt){Param1=0, Param2=0}
      mask prompts: Param1 "XTable:"; Param2 "YTable:"
      settings: AttributesFormatString=IntplVarXY (sX, uY)
      mask Help: <p>This block was generated automatically by the Legacy Code Tool. For detailed help on this tool, call<a href="matlab:legacy_code('help')"> legacy_code('help')</a>.</p>
      mask Display:
      | %port_label('input',1,'u');
      | %port_label('output',1,'(u16)');
      | 
      | Xx = [0, .9];
      | Xy = [.05, .05];
      | Yx = [.45, .45];
      | Yy = [.05, .9];
      | 
      | px = [0, .3, .4, .6, .7, .9];
      | py = [.15, .15, .2, .5, .6, .65];
      | plot(Xx,Xy, Yx,Yy, px,py)
  IntplVarXY_u16_u16Xu16Y_Cnt : S-Function  FunctionName=IntplVarXY_u16_u16Xu16Y_Cnt  Parameters=Param1,Param2  EnableBusSupport=off  mask(IntplVarXY_u16_u16Xu16Y_Cnt){Param1=0, Param2=0}
      mask prompts: Param1 "XTable:"; Param2 "YTable:"
      settings: AttributesFormatString=IntplVarXY (uX, uY)
      mask Help: <p>This block was generated automatically by the Legacy Code Tool. For detailed help on this tool, call<a href="matlab:legacy_code('help')"> legacy_code('help')</a>.</p>
      mask Display:
      | %port_label('input',1,'u');
      | %port_label('output',1,'(u16)');
      | 
      | Xx = [0.1, .9];
      | Xy = [0.1, 0.1];
      | Yx = [0.1, 0.1];
      | Yy = [0.1, .9];
      | 
      | px = [0.1, .2, .3, .4, .5, .6, .8];
      | py = [0.1,  0.4, .6, .7, .75, .78, .8];
      | plot(Xx,Xy, Yx,Yy, px,py)

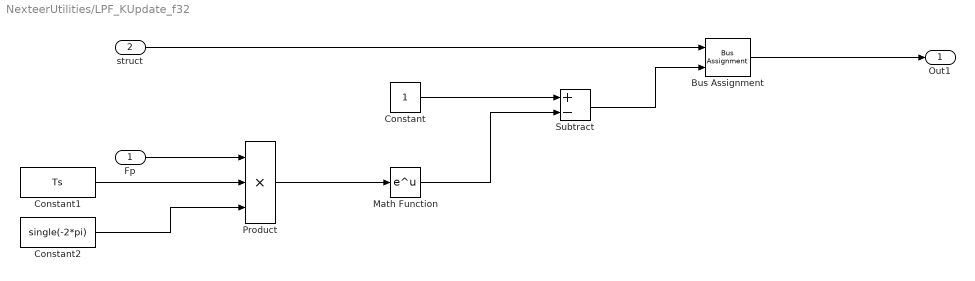
== system NexteerUtilities/LPF_KUpdate_f32 ==
  Fp : Inport  OutDataTypeStr=single
  struct : Inport  Port=2  OutDataTypeStr=Bus: LPF32KSV_Str
  Bus Assignment : BusAssignment  AssignedSignals=K_Uls_f32
  Constant : Constant  OutDataTypeStr=single
  Constant1 : Constant  Value=Ts  OutDataTypeStr=single
  Constant2 : Constant  Value=single(-2*pi)  OutDataTypeStr=single
  Math Function : Math  SaturateOnIntegerOverflow=on
  Product : Product  Inputs=3
  Subtract : Sum  Inputs=+-
  Out1 : Outport  OutDataTypeStr=Bus: LPF32KSV_Str
  wires:
  Constant/1 -> Subtract/1
  Math Function/1 -> Subtract/2
  Constant1/1 -> Product/2
  Fp/1 -> Product/1
  Product/1 -> Math Function/1
  struct/1 -> Bus Assignment/1
  Subtract/1 -> Bus Assignment/2
  Bus Assignment/1 -> Out1/1
  Constant2/1 -> Product/3

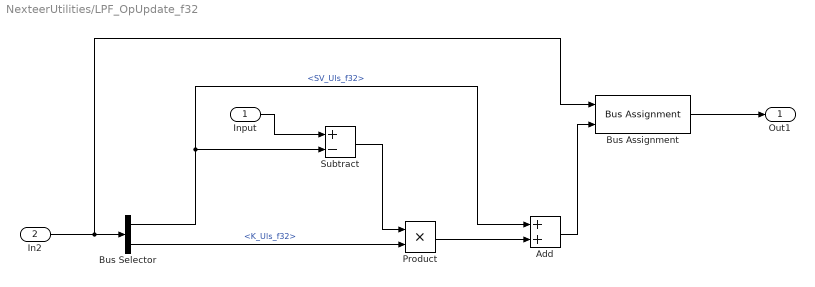
== system NexteerUtilities/LPF_OpUpdate_f32 ==
  Input : Inport
  In2 : Inport  Port=2  OutDataTypeStr=Bus: LPF32KSV_Str
  Add : Sum
  Bus Assignment : BusAssignment  AssignedSignals=SV_Uls_f32
  Bus Selector : BusSelector  OutputSignals=SV_Uls_f32,K_Uls_f32
  Product : Product
  Subtract : Sum  Inputs=+-
  Out1 : Outport  OutDataTypeStr=Bus: LPF32KSV_Str
  wires:
  In2/1 -> Bus Assignment/1, Bus Selector/1
  Bus Selector/2 -> Product/2  "<K_Uls_f32>"
  Bus Selector/1 -> Add/1, Subtract/2  "<SV_Uls_f32>"
  Input/1 -> Subtract/1
  Subtract/1 -> Product/1
  Product/1 -> Add/2
  Add/1 -> Bus Assignment/2
  Bus Assignment/1 -> Out1/1

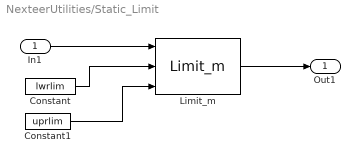
== system NexteerUtilities/Static_Limit ==
  In1 : Inport
  Constant : Constant  Value=lwrlim
  Constant1 : Constant  Value=uprlim
  Limit_m : S-Function  FunctionName=Limit_m  EnableBusSupport=off
      mask Display:
      | port_label('input',1,'U');
      | port_label('input',2,'Lwr Limit');
      | port_label('input',3,'Upr Limit');
      | port_label('output',1,'Y');
  Out1 : Outport
  wires:
  Limit_m/1 -> Out1/1
  In1/1 -> Limit_m/1
  Constant/1 -> Limit_m/2
  Constant1/1 -> Limit_m/3

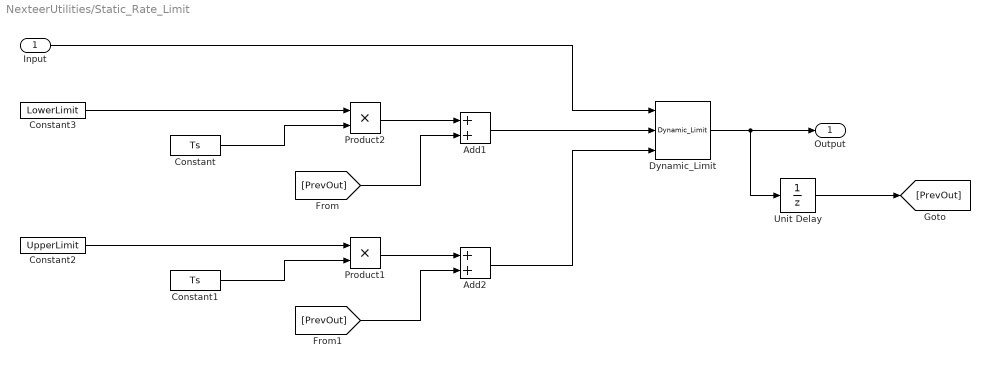
== system NexteerUtilities/Static_Rate_Limit ==
  Input : Inport
  Add1 : Sum
  Add2 : Sum
  Constant : Constant  Value=Ts
  Constant1 : Constant  Value=Ts
  Constant2 : Constant  Value=UpperLimit
  Constant3 : Constant  Value=LowerLimit
  Dynamic_Limit : NexteerUtilities/Dynamic_Limit
  Product1 : Product
  Product2 : Product
  Unit Delay : UnitDelay  SampleTime=-1
  Output : Outport
  wires:
  Dynamic_Limit/1 -> Output/1, Unit Delay/1
  Input/1 -> Dynamic_Limit/1
  Constant/1 -> Product2/2
  Constant3/1 -> Product2/1
  Product2/1 -> Add1/1
  Unit Delay/1 -> [PrevOut]
  [PrevOut] -> Add1/2
  Add1/1 -> Dynamic_Limit/2
  Constant1/1 -> Product1/2
  Constant2/1 -> Product1/1
  Product1/1 -> Add2/1
  [PrevOut] -> Add2/2
  Add2/1 -> Dynamic_Limit/3
